simulink model "DC_Motor"  (R2019a)
settings: Solver=VariableStepAuto  StartTime=0.0  StopTime=10.0  RelTol=1e-3
model workspace (MATLAB code in the model file):
  | L = 1;
  | R=1;
  | K_b=1;
  | J=1;
  | K_f=1;
  | K_m=1;
settings Model: Creator=manfred  LastModifiedBy=manfred

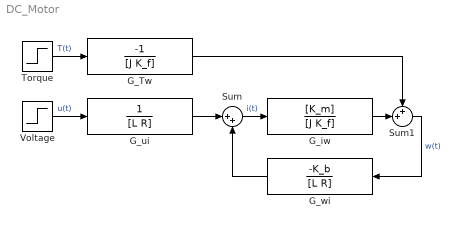
== system DC_Motor ==
  G_Tw : TransferFcn  Numerator=-1  Denominator=[J K_f]
  G_iw : TransferFcn  Numerator=[K_m]  Denominator=[J K_f]  ContinuousStateAttributes='w(t)'
  G_ui : TransferFcn  Numerator=1  Denominator=[L R]
  G_wi : TransferFcn  Numerator=-K_b  Denominator=[L R]
  Sum : Sum  Inputs=|++
  Sum1 : Sum  Inputs=++|
  Torque : Step  SampleTime=0
  Voltage : Step  SampleTime=0
  wires:
  G_wi/1 -> Sum/2
  Sum/1 -> G_iw/1  "i(t)"
  G_iw/1 -> Sum1/2
  G_Tw/1 -> Sum1/1
  G_ui/1 -> Sum/1
  Voltage/1 -> G_ui/1  "u(t)"
  Torque/1 -> G_Tw/1  "T(t)"
  Sum1/1 -> G_wi/1  "w(t)"
